simulink model "Vergleich_Regler_nach_Ziegler_Nichols"  (R2016a)
settings: Solver=ode3  StartTime=0.0  StopTime=100  FixedStep=0.1  RelTol=1e-3
settings Model: Creator=gregor  LastModifiedBy=gregor
settings DataIOCC: LimitDataPoints=on  SaveFormat=Array  SignalLoggingSaveFormat=ModelDataLogs  SaveState=on
settings OptimizationCC: ExpressionDepthLimit=2147483647  InitFltsAndDblsToZero=on
settings DebuggingCC: SaveWithParameterizedLinksMsg=none  UnderspecifiedInitializationDetection=Classic  MergeDetectMultiDrivingBlocksExec=none  SignalResolutionControl=TryResolveAllWithWarning  SolverPrmCheckMsg=warning  MultiTaskDSMMsg=warning  MultiTaskCondExecSysMsg=none  FcnCallInpInsideContextMsg=UseLocalSettings  StateNameClashWarn=warning
settings HardwareCC: ProdBitPerPointer=32  ProdLargestAtomicFloat=None  ProdIntDivRoundTo=Undefined  ProdEndianess=Unspecified  ProdWordSize=32  ProdHWDeviceType=32-bit Generic
settings ModelReferenceCC: PropagateSignalLabelsOutOfModel=off
settings GRTTargetCC: TargetFcnLib=ansi_tfl_tmw.mat  GeneratePreprocessorConditionals=Use local settings  CombineOutputUpdateFcns=off  GRTInterface=on
settings ConfigComp: CovModelRefEnable=Off

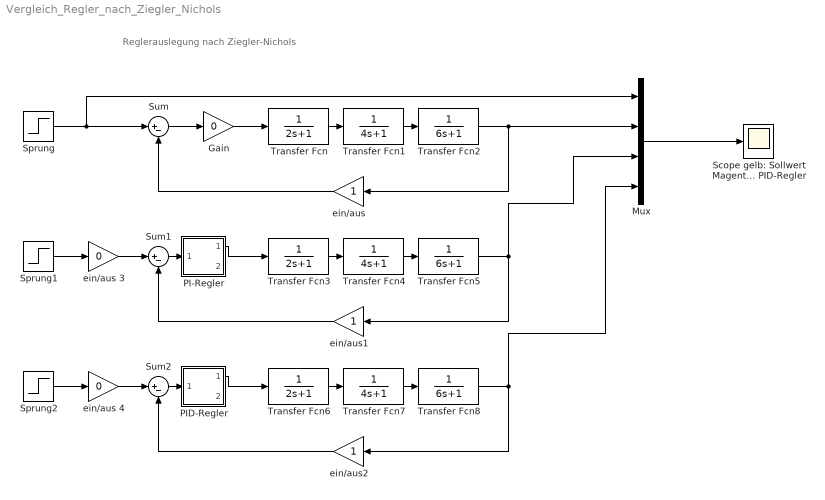
== system Vergleich_Regler_nach_Ziegler_Nichols ==
  note: Reglerauslegung nach Ziegler-Nichols
  Gain : Gain  Gain=0
  Mux : Mux
  PI-Regler : Subsystem  mask{P=1, I=12.6*0.85}
      mask prompts: P "Verstärkung (K)"; I "Nachlaufzeit (T_n)"
      mask help:
      | PI-Regler:
      |
      | G_R(s) = K(1 + 1/(s*T_n))
      mask Help:
      | PI-Regler:
      | 
      | G_R(s) = K(1 + 1/(s*T_n))
      mask Display: disp('PI');
  PID-Regler : Subsystem  mask{P=1, I=1, D=1}
      mask prompts: P "Verstärkung (K)"; I "Nachlaufzeit (T_n)"; D "Vorhaltzeit (T_v)"
      mask help:
      | PID-Regler:
      |
      | F_R(s) = K(1 + 1/(s*T_n) + T_v*s)
      mask Help:
      | PID-Regler:
      | 
      | F_R(s) = K(1 + 1/(s*T_n) + T_v*s)
      mask Display: disp('PID');
  Scope gelb: Sollwert Magenta: P-Regler Cyan: PI-Regler Rot: PID-Regler : Scope
  Sprung : Step  SampleTime=0
  Sprung1 : Step  SampleTime=0
  Sprung2 : Step  SampleTime=0
  Sum : Sum  Inputs=|+-
  Sum1 : Sum  Inputs=|+-
  Sum2 : Sum  Inputs=|+-
  Transfer Fcn : TransferFcn  Numerator=1  Denominator=[2 1]
  Transfer Fcn1 : TransferFcn  Denominator=[4 1]
  Transfer Fcn2 : TransferFcn  Denominator=[6 1]
  Transfer Fcn3 : TransferFcn  Numerator=1  Denominator=[2 1]
  Transfer Fcn4 : TransferFcn  Denominator=[4 1]
  Transfer Fcn5 : TransferFcn  Denominator=[6 1]
  Transfer Fcn6 : TransferFcn  Numerator=1  Denominator=[2 1]
  Transfer Fcn7 : TransferFcn  Denominator=[4 1]
  Transfer Fcn8 : TransferFcn  Denominator=[6 1]
  ein/aus : Gain
  ein/aus 3 : Gain  Gain=0
  ein/aus 4 : Gain  Gain=0
  ein/aus1 : Gain
  ein/aus2 : Gain
  wires:
  Transfer Fcn/1 -> Transfer Fcn1/1
  Transfer Fcn1/1 -> Transfer Fcn2/1
  Mux/1 -> Scope gelb: Sollwert Magenta: P-Regler Cyan: PI-Regler Rot: PID-Regler/1
  Sum/1 -> Gain/1
  Transfer Fcn2/1 -> ein/aus/1, Mux/2
  ein/aus/1 -> Sum/2
  Transfer Fcn3/1 -> Transfer Fcn4/1
  Transfer Fcn4/1 -> Transfer Fcn5/1
  Sum1/1 -> PI-Regler/1(In_1)
  Transfer Fcn5/1 -> ein/aus1/1, Mux/3
  PI-Regler/1(Out_1) -> Transfer Fcn3/1
  ein/aus1/1 -> Sum1/2
  Transfer Fcn6/1 -> Transfer Fcn7/1
  Transfer Fcn7/1 -> Transfer Fcn8/1
  Sum2/1 -> PID-Regler/1(In_1)
  Transfer Fcn8/1 -> ein/aus2/1, Mux/4
  PID-Regler/1(Out_1) -> Transfer Fcn6/1
  ein/aus2/1 -> Sum2/2
  Gain/1 -> Transfer Fcn/1
  Sprung/1 -> Mux/1, Sum/1
  Sprung1/1 -> ein/aus 3/1
  ein/aus 3/1 -> Sum1/1
  Sprung2/1 -> ein/aus 4/1
  ein/aus 4/1 -> Sum2/1

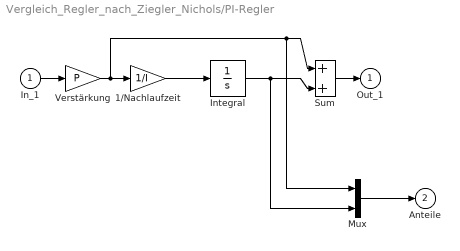
== system Vergleich_Regler_nach_Ziegler_Nichols/PI-Regler ==
  In_1 : Inport
  1/Nachlaufzeit : Gain  Gain=1/I  SaturateOnIntegerOverflow=on  OutDataTypeStr=Inherit: Same as input  ParamDataTypeStr=Inherit: Same as input
  Integral : TransferFcn  Denominator=[1 0]
  Mux : Mux  Inputs=2
  Sum : Sum  SaturateOnIntegerOverflow=on  InputSameDT=on  OutDataTypeStr=Inherit: Same as first input
  Verstärkung : Gain  Gain=P  SaturateOnIntegerOverflow=on  OutDataTypeStr=Inherit: Same as input  ParamDataTypeStr=Inherit: Same as input
  Out_1 : Outport  InitialOutput=0
  Anteile : Outport  Port=2  InitialOutput=0
  wires:
  Integral/1 -> Sum/2, Mux/2
  Sum/1 -> Out_1/1
  In_1/1 -> Verstärkung/1
  Verstärkung/1 -> 1/Nachlaufzeit/1, Mux/1, Sum/1
  1/Nachlaufzeit/1 -> Integral/1
  Mux/1 -> Anteile/1

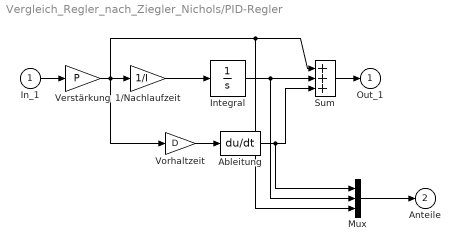
== system Vergleich_Regler_nach_Ziegler_Nichols/PID-Regler ==
  In_1 : Inport
  1/Nachlaufzeit : Gain  Gain=1/I  SaturateOnIntegerOverflow=on  OutDataTypeStr=Inherit: Same as input  ParamDataTypeStr=Inherit: Same as input
  Ableitung : Derivative
  Integral : TransferFcn  Denominator=[1 0]
  Mux : Mux  Inputs=3
  Sum : Sum  Inputs=+++  SaturateOnIntegerOverflow=on  InputSameDT=on  OutDataTypeStr=Inherit: Same as first input
  Verstärkung : Gain  Gain=P  SaturateOnIntegerOverflow=on  OutDataTypeStr=Inherit: Same as input  ParamDataTypeStr=Inherit: Same as input
  Vorhaltzeit : Gain  Gain=D  SaturateOnIntegerOverflow=on  OutDataTypeStr=Inherit: Same as input  ParamDataTypeStr=Inherit: Same as input
  Out_1 : Outport  InitialOutput=0
  Anteile : Outport  Port=2  InitialOutput=0
  wires:
  Integral/1 -> Sum/2, Mux/2
  Ableitung/1 -> Sum/3, Mux/1
  Sum/1 -> Out_1/1
  Vorhaltzeit/1 -> Ableitung/1
  In_1/1 -> Verstärkung/1
  Verstärkung/1 -> 1/Nachlaufzeit/1, Vorhaltzeit/1, Sum/1, Mux/3
  1/Nachlaufzeit/1 -> Integral/1
  Mux/1 -> Anteile/1
